simulink model "lab5pq3noisesim"  (R2018a)
settings: Solver=VariableStepAuto  StartTime=0.0  StopTime=10.0  RelTol=1e-3
libraries: dspfdesign x1
settings Model: Creator=ja_ping  LastModifiedBy=ja_ping

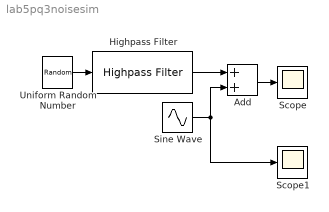
== system lab5pq3noisesim ==
  Add : Sum
  Highpass Filter : dspfdesign/Highpass Filter  FilterType=IIR  DesignForMinimumOrder=on  FilterOrder=50  StopbandFrequency=3600  PassbandFrequency=3800  StopbandAttenuation=60  PassbandRipple=1  InheritSampleRate=off  SampleRate=8000  SimulateUsing=Interpreted execution  roundingMode=Floor  coeffsDataTypeStr=fixdt(1,16)
      settings: SourceProductName=DSP System Toolbox
  Scope : Scope
  Scope1 : Scope
  Sine Wave : Sin  Frequency=100  SampleTime=1/8000
  Uniform Random Number : UniformRandomNumber  Minimum=-5  Maximum=5  SampleTime=1/8000
  wires:
  Uniform Random Number/1 -> Highpass Filter/1
  Highpass Filter/1 -> Add/1
  Sine Wave/1 -> Scope1/1, Add/2
  Add/1 -> Scope/1
